simulink model "roverSim"  (R2022b)
settings: Solver=FixedStepAuto  StartTime=0.0  StopTime=86400  FixedStep=1  RelTol=1e-3
values from neighbouring files (symbols this model uses):
  rv = rover    [config.m]
undefined symbols (not defined in the file or in its folder): modes
settings Model: SimulationMode=accelerator  Creator=HelloWorld  LastModifiedBy=HelloWorld

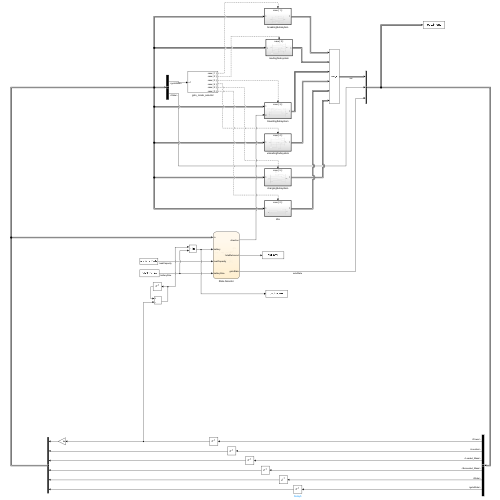
[thumbnail: Simulink's stored preview of the top-level diagram]
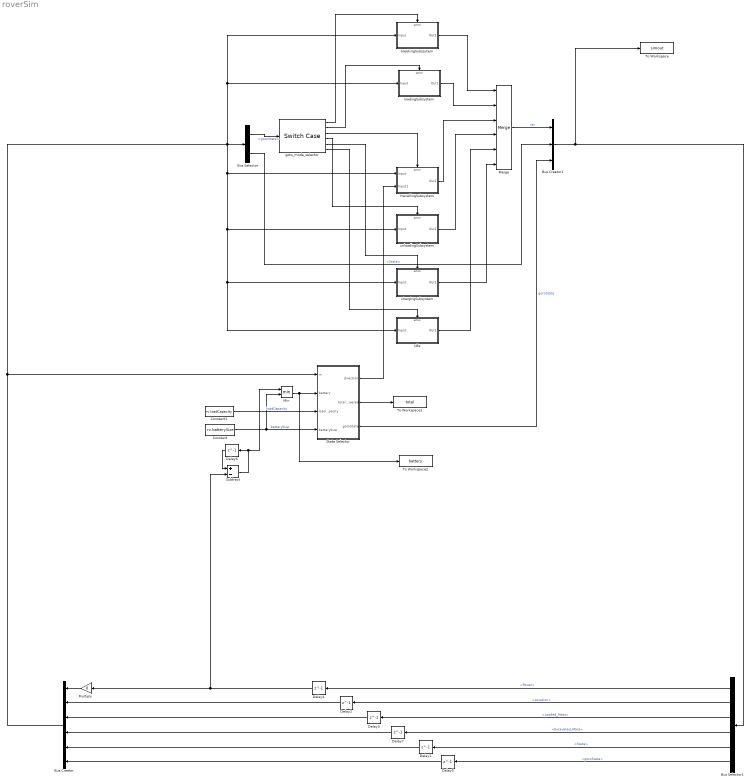
== system roverSim ==
  Bus Creator : BusCreator  Inputs=6  OutDataTypeStr=Bus: curState
      settings: InheritFromInputs=off
  Bus Creator1 : BusCreator  Inputs=3
  Bus Selector : BusSelector  OutputSignals=gotoState,State
  Bus Selector1 : BusSelector  OutputSignals=var.Power,var.Location,var.Loaded_Mass,var.Excavated_Mass,State,gotoState
  Constant : Constant  Value=rv.batterySize
  Constant1 : Constant  Value=rv.loadCapacity
  Delay1 : Delay  DelayLength=1  InitialCondition=int8(modes.breaking)
  Delay{2..4,7} (4 alike) : Delay  DelayLength=1  InitialCondition=0
  Delay5 : Delay  DelayLength=1  InitialCondition=int8(modes.idle)
  Delay6 : Delay  DelayLength=1  InitialCondition=rv.batterySize
  Idle : Subsystem  TreatAsAtomicUnit=on
  Merge : Merge  Inputs=6
  Min : MinMax  Inputs=2
  Multiply : Gain  Gain=0
  State Selector : Stateflow chart  TreatAsAtomicUnit=on
  Subtract : Sum  Inputs=+-
  To Workspace : ToWorkspace  VariableName=simout  SaveFormat=Timeseries  SampleTime=-1
  To Workspace1 : ToWorkspace  VariableName=total  SampleTime=-1
      settings: Save2DSignal=2-D array (concatenate along first dimension)
  To Workspace2 : ToWorkspace  VariableName=battery  SampleTime=-1
      settings: Save2DSignal=2-D array (concatenate along first dimension)
  breakingSubssytem : Subsystem  TreatAsAtomicUnit=on
  chargingSubsystem : Subsystem  TreatAsAtomicUnit=on
  goto_mode_selector : SwitchCase  CaseConditions={1, 2, 3, 4, 5, 0}  ShowDefaultCase=off
  loadingSubsystem : Subsystem  TreatAsAtomicUnit=on
  travellingSubsystem : Subsystem  TreatAsAtomicUnit=on
  unloadingSubsystem : Subsystem  TreatAsAtomicUnit=on
  wires:
  goto_mode_selector/1 -> breakingSubssytem/Action
  goto_mode_selector/2 -> loadingSubsystem/Action
  goto_mode_selector/3 -> travellingSubsystem/Action
  breakingSubssytem/1(Out1) -> Merge/1
  loadingSubsystem/1(Out1) -> Merge/2
  travellingSubsystem/1(Out1) -> Merge/3
  Bus Selector/1 -> goto_mode_selector/1  "<gotoState>"
  Bus Selector1/1 -> Delay4/1  "<Power>"
  Bus Selector1/2 -> Delay2/1  "<Location>"
  Bus Selector1/3 -> Delay3/1  "<Loaded_Mass>"
  Bus Selector1/5 -> Delay1/1  "<State>"
  Bus Selector1/6 -> Delay5/1  "<gotoState>"
  Bus Creator/1 -> breakingSubssytem/1(Input), loadingSubsystem/1(Input), Idle/1(Input), chargingSubsystem/1(Input), unloadingSubsystem/1(Input), travellingSubsystem/1(Input), Bus Selector/1, State Selector/1(in)
  Delay1/1 -> Bus Creator/5
  Delay2/1 -> Bus Creator/2
  Delay3/1 -> Bus Creator/3
  Delay4/1 -> Multiply/1, Subtract/2
  Delay5/1 -> Bus Creator/6
  Multiply/1 -> Bus Creator/1
  Bus Creator1/1 -> To Workspace/1, Bus Selector1/1
  Merge/1 -> Bus Creator1/1  "var"
  Bus Selector/2 -> Bus Creator1/2  "<State>"
  State Selector/3(gotoState) -> Bus Creator1/3  "gotoState"
  State Selector/1(direction) -> travellingSubsystem/2(Input1)
  goto_mode_selector/4 -> unloadingSubsystem/Action
  unloadingSubsystem/1(Out1) -> Merge/4
  Idle/1(Out1) -> Merge/5
  State Selector/2(totalDelivered) -> To Workspace1/1
  Constant/1 -> Min/2, State Selector/4(batterySize)  "batterySize"
  goto_mode_selector/5 -> chargingSubsystem/Action
  goto_mode_selector/6 -> Idle/Action
  chargingSubsystem/1(Out1) -> Merge/6
  Constant1/1 -> State Selector/3(loadCapacity)  "loadCapacity"
  Subtract/1 -> Min/1, Delay6/1
  Delay6/1 -> Subtract/1
  Min/1 -> To Workspace2/1, State Selector/2(battery)
  Bus Selector1/4 -> Delay7/1  "<Excavated_Mass>"
  Delay7/1 -> Bus Creator/4

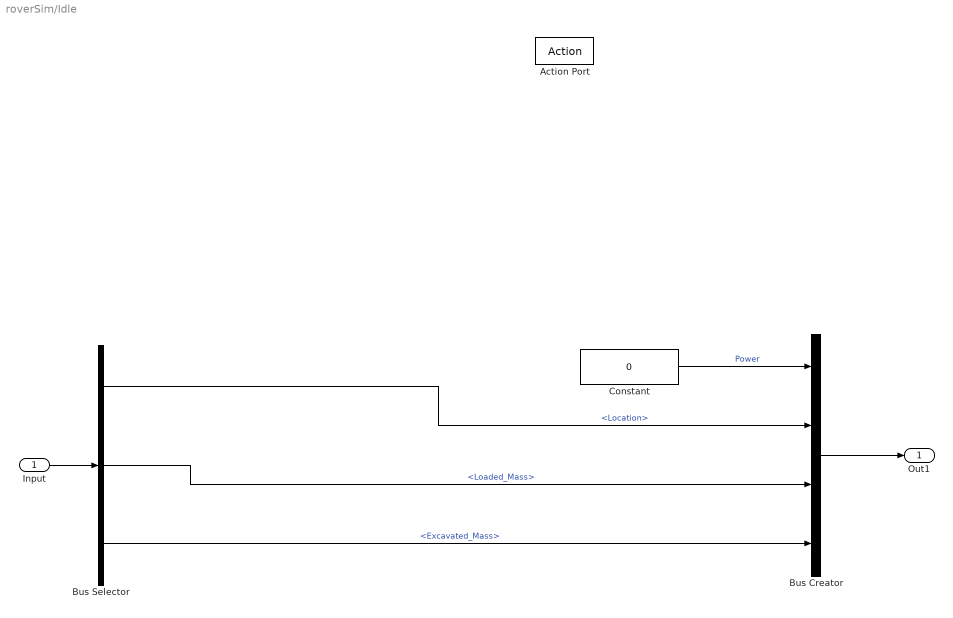
== system roverSim/Idle ==
  Input : Inport  OutDataTypeStr=Bus: curState
  Action Port : ActionPort  ActionPortLabel=case [ 0 ]:
  Bus Creator : BusCreator  Inputs=4
  Bus Selector : BusSelector  OutputSignals=Location,Loaded_Mass,Excavated_Mass
  Constant : Constant  Value=0
  Out1 : Outport  LockScale=on
  wires:
  Input/1 -> Bus Selector/1
  Constant/1 -> Bus Creator/1  "Power"
  Bus Creator/1 -> Out1/1
  Bus Selector/3 -> Bus Creator/4  "<Excavated_Mass>"
  Bus Selector/2 -> Bus Creator/3  "<Loaded_Mass>"
  Bus Selector/1 -> Bus Creator/2  "<Location>"

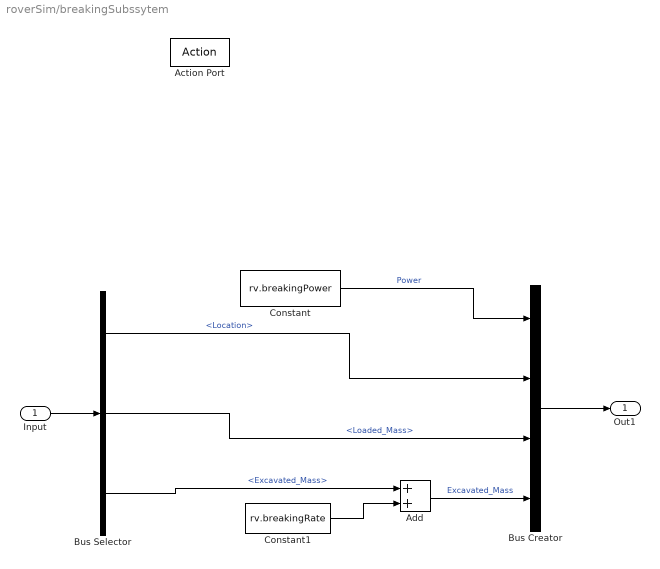
== system roverSim/breakingSubssytem ==
  Input : Inport  OutDataTypeStr=Bus: curState
  Action Port : ActionPort  ActionPortLabel=case [ 1 ]:
  Add : Sum
  Bus Creator : BusCreator  Inputs=4
  Bus Selector : BusSelector  OutputSignals=Location,Loaded_Mass,Excavated_Mass
  Constant : Constant  Value=rv.breakingPower
  Constant1 : Constant  Value=rv.breakingRate
  Out1 : Outport  LockScale=on
  wires:
  Input/1 -> Bus Selector/1
  Constant1/1 -> Add/2
  Constant/1 -> Bus Creator/1  "Power"
  Bus Selector/1 -> Bus Creator/2  "<Location>"
  Bus Selector/2 -> Bus Creator/3  "<Loaded_Mass>"
  Bus Selector/3 -> Add/1  "<Excavated_Mass>"
  Add/1 -> Bus Creator/4  "Excavated_Mass"
  Bus Creator/1 -> Out1/1

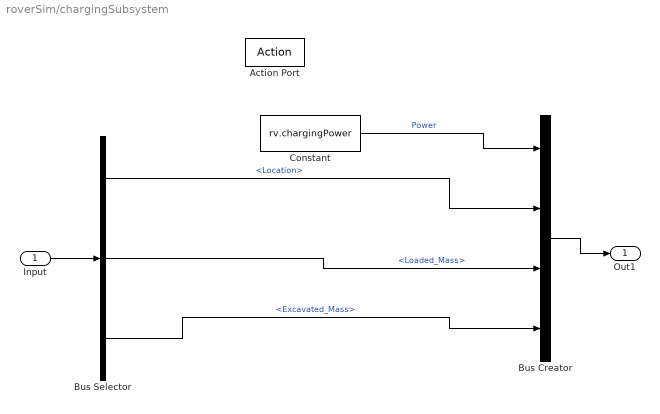
== system roverSim/chargingSubsystem ==
  Input : Inport  OutDataTypeStr=Bus: curState
  Action Port : ActionPort  ActionPortLabel=case [ 5 ]:
  Bus Creator : BusCreator  Inputs=4
  Bus Selector : BusSelector  OutputSignals=Location,Loaded_Mass,Excavated_Mass
  Constant : Constant  Value=rv.chargingPower
  Out1 : Outport  LockScale=on
  wires:
  Input/1 -> Bus Selector/1
  Constant/1 -> Bus Creator/1  "Power"
  Bus Selector/1 -> Bus Creator/2  "<Location>"
  Bus Creator/1 -> Out1/1
  Bus Selector/3 -> Bus Creator/4  "<Excavated_Mass>"
  Bus Selector/2 -> Bus Creator/3  "<Loaded_Mass>"

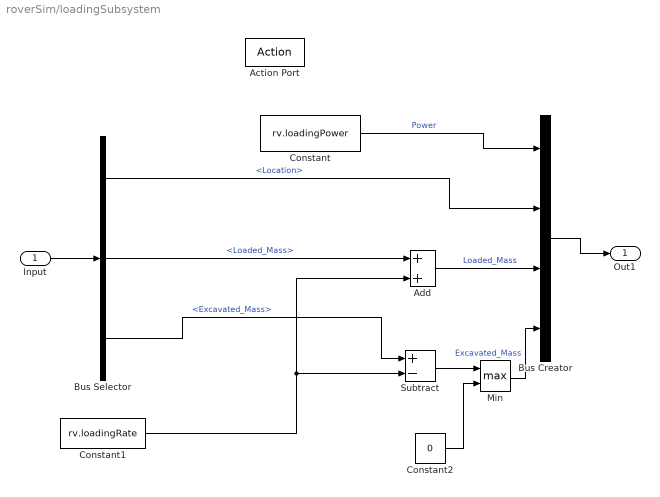
== system roverSim/loadingSubsystem ==
  Input : Inport  OutDataTypeStr=Bus: curState
  Action Port : ActionPort  ActionPortLabel=case [ 2 ]:
  Add : Sum
  Bus Creator : BusCreator  Inputs=4
  Bus Selector : BusSelector  OutputSignals=Location,Loaded_Mass,Excavated_Mass
  Constant : Constant  Value=rv.loadingPower
  Constant1 : Constant  Value=rv.loadingRate
  Constant2 : Constant  Value=0
  Min : MinMax  Function=max  Inputs=2
  Subtract : Sum  Inputs=+-
  Out1 : Outport  LockScale=on
  wires:
  Input/1 -> Bus Selector/1
  Constant/1 -> Bus Creator/1  "Power"
  Bus Selector/1 -> Bus Creator/2  "<Location>"
  Bus Creator/1 -> Out1/1
  Add/1 -> Bus Creator/3  "Loaded_Mass"
  Bus Selector/2 -> Add/1  "<Loaded_Mass>"
  Bus Selector/3 -> Subtract/1  "<Excavated_Mass>"
  Constant1/1 -> Subtract/2, Add/2
  Subtract/1 -> Min/1
  Min/1 -> Bus Creator/4  "Excavated_Mass"
  Constant2/1 -> Min/2

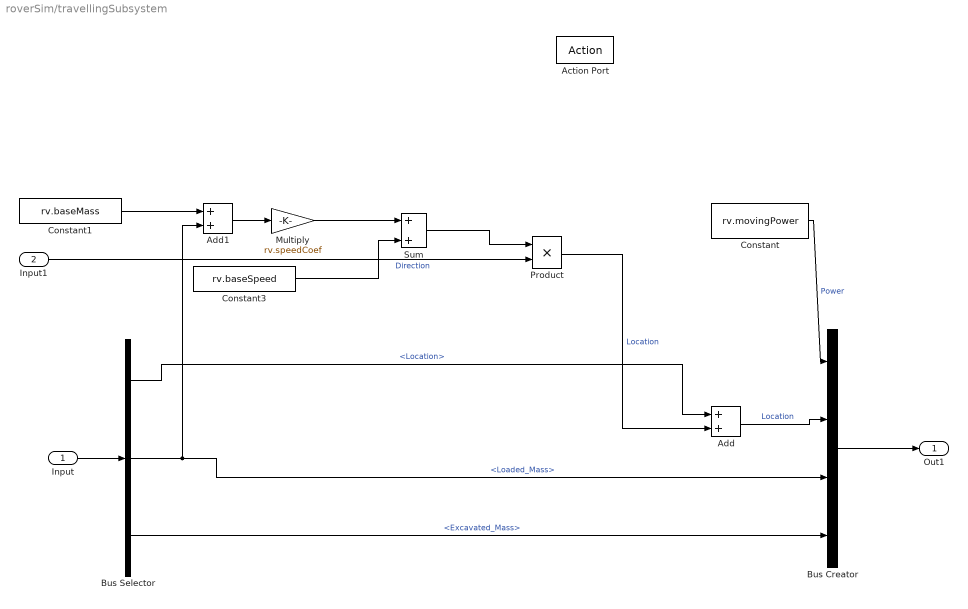
== system roverSim/travellingSubsystem ==
  Input : Inport  OutDataTypeStr=Bus: curState
  Input1 : Inport  Port=2
  Action Port : ActionPort  ActionPortLabel=case [ 3 ]:
  Add : Sum
  Add1 : Sum
  Bus Creator : BusCreator  Inputs=4
  Bus Selector : BusSelector  OutputSignals=Location,Loaded_Mass,Excavated_Mass
  Constant : Constant  Value=rv.movingPower
  Constant1 : Constant  Value=rv.baseMass
  Constant3 : Constant  Value=rv.baseSpeed
  Multiply : Gain  Gain=rv.speedCoef
  Product : Product
  Sum : Sum
  Out1 : Outport  LockScale=on
  wires:
  Input/1 -> Bus Selector/1
  Constant/1 -> Bus Creator/1  "Power"
  Bus Creator/1 -> Out1/1
  Constant1/1 -> Add1/1
  Add1/1 -> Multiply/1
  Multiply/1 -> Sum/1
  Constant3/1 -> Sum/2
  Bus Selector/1 -> Add/1  "<Location>"
  Bus Selector/3 -> Bus Creator/4  "<Excavated_Mass>"
  Bus Selector/2 -> Bus Creator/3, Add1/2  "<Loaded_Mass>"
  Sum/1 -> Product/1
  Product/1 -> Add/2  "Location"
  Add/1 -> Bus Creator/2  "Location"
  Input1/1 -> Product/2  "Direction"

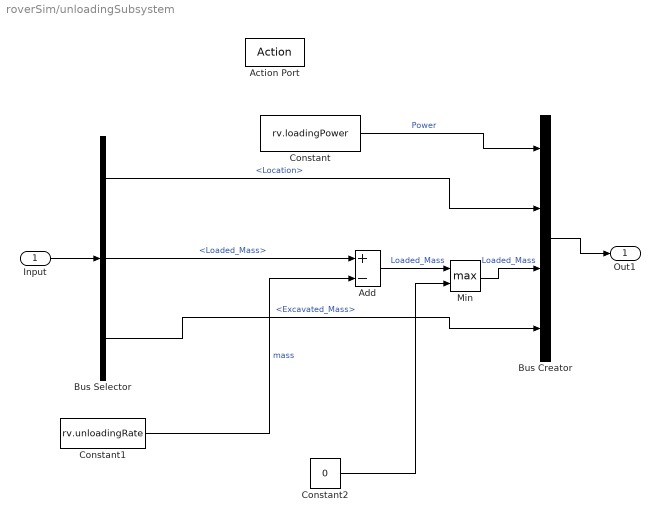
== system roverSim/unloadingSubsystem ==
  Input : Inport  OutDataTypeStr=Bus: curState
  Action Port : ActionPort  ActionPortLabel=case [ 4 ]:
  Add : Sum  Inputs=+-
  Bus Creator : BusCreator  Inputs=4
  Bus Selector : BusSelector  OutputSignals=Location,Loaded_Mass,Excavated_Mass
  Constant : Constant  Value=rv.loadingPower
  Constant1 : Constant  Value=rv.unloadingRate
  Constant2 : Constant  Value=0
  Min : MinMax  Function=max  Inputs=2
  Out1 : Outport  LockScale=on
  wires:
  Input/1 -> Bus Selector/1
  Constant/1 -> Bus Creator/1  "Power"
  Bus Selector/1 -> Bus Creator/2  "<Location>"
  Bus Creator/1 -> Out1/1
  Bus Selector/2 -> Add/1  "<Loaded_Mass>"
  Bus Selector/3 -> Bus Creator/4  "<Excavated_Mass>"
  Constant1/1 -> Add/2  "mass"
  Constant2/1 -> Min/2
  Add/1 -> Min/1  "Loaded_Mass"
  Min/1 -> Bus Creator/3  "Loaded_Mass"

== stateflow chart roverSim/State Selector ==
  state Done
    gotoState=int8(modes.idle);
  state Charging
    entry, during:
    gotoState=int8(modes.charging);
  state Init
    gotoState=int8(modes.idle);
    direction=1;
    totalDelivered=0;
    load=0;
  state Idle
    gotoState=int8(modes.idle);
  state Excavate
    gotoState=int8(modes.breaking);
  state Load
    gotoState=int8(modes.loading);
  state MoveToPit
    gotoState=int8(modes.travelling);
    direction=-1;
  state MoveToSite
    gotoState=int8(modes.travelling);
    direction=1;
    load=in.Loaded_Mass;
  state Unload
    gotoState=int8(modes.unloading);
  Charging -> Done [order 2] : [totalDelivered>400 & battery/batterySize>0.99]
  (default) -> Init
  Excavate -> Charging [order 1] : [totalDelivered>400]
  Excavate -> Charging [order 3] : [battery/batterySize<0.3]
  Init -> Idle
  Idle -> Excavate : [in.Excavated_Mass <= loadCapacity]
  Charging -> Excavate [order 1] : [battery/batterySize>0.99 & totalDelivered<400]
  MoveToPit -> Excavate : [in.Location <=0.1]
  Excavate -> Load [order 2] : [in.Excavated_Mass> loadCapacity && battery/batterySize>0.4]
  Unload -> MoveToPit : [in.Loaded_Mass <=0]
      | {totalDelivered=totalDelivered+load;}
  Load -> MoveToSite : [in.Loaded_Mass > loadCapacity]
  MoveToSite -> Unload : [in.Location >= 500]
  data: direction output; totalDelivered output double; in input Bus: curState; battery input; gotoState output int8; load local; loadCapacity input; batterySize input
